simulink model "PoolofAdaptiveoscillatorsThree"  (R2019b)
settings: Solver=FixedStepAuto  StartTime=0.0  StopTime=t_sim  FixedStep=tsamp  MaxStep=0.01  RelTol=1e-3
values from neighbouring files (symbols this model uses):
  alpha_0_init = 0.01    [PoolofAdaptiveOscillatorsThree.m]
  alpha_init = 0    [PoolofAdaptiveOscillatorsThree.m]
  eta = 2    [AO_Oscillators.m]    (also in PoolofAdaptiveOscillatorsThree.m = 1)
  omega_init = 0    [PoolofAdaptiveOscillatorsThree.m]
  phi_init = 0    [PoolofAdaptiveOscillatorsThree.m]
  tsamp = T/100    (= 0.0125)    [AO_Oscillators.m]    (also in PoolofAdaptiveOscillatorsThree.m = 0.00625)
  v_omega = 13    [AO_Oscillators.m]    (also in PoolofAdaptiveOscillatorsThree.m = 2)
  v_phi = sqrt(24.2*v_omega)    [AO_Oscillators.m]    (also in PoolofAdaptiveOscillatorsThree.m = 2)
settings Model: Creator=dell  LastModifiedBy=dell

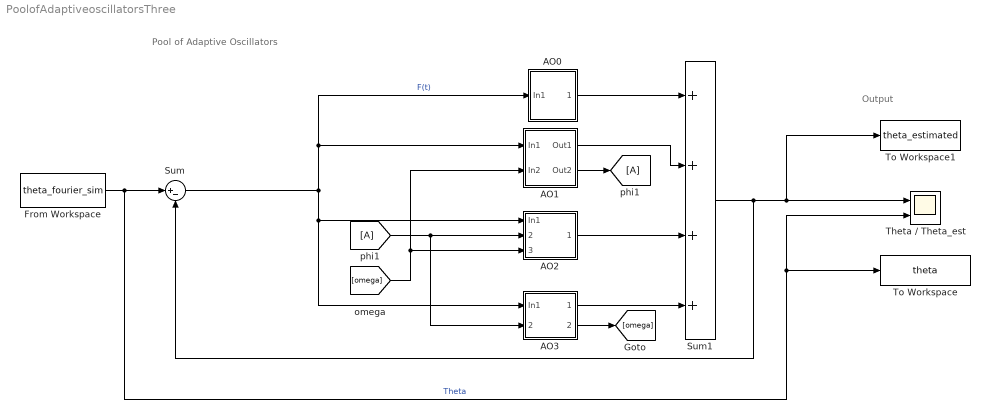
== system PoolofAdaptiveoscillatorsThree ==
  note: Pool of Adaptive Oscillators
  note: Output
  AO0 : Subsystem
      mask Display: image('F:\Masters\Thesis\Scripts\Images\integ.png'); % Use "Edit Image" on toolstrip to change.
  AO1 : Subsystem
      mask Display: image('F:\Masters\Thesis\Scripts\Images\ac symbol.png'); % Use "Edit Image" on toolstrip to change.
  AO2 : Subsystem
      mask Display: image('F:\Masters\Thesis\Scripts\Images\ac symbol.png'); % Use "Edit Image" on toolstrip to change.
  AO3 : Subsystem
      mask Display: image('F:\Masters\Thesis\Scripts\Images\ac symbol.png'); % Use "Edit Image" on toolstrip to change.
  From Workspace : FromWorkspace  VariableName=theta_fourier_sim  SampleTime=tsamp  Interpolate=off  OutputAfterFinalValue=Holding final value
  Sum : Sum  Inputs=|+-
  Sum1 : Sum  Inputs=4
  "Theta / Theta_est " : Scope  NumInputPorts=2
  To Workspace : ToWorkspace  VariableName=theta  SaveFormat=Timeseries  SampleTime=-1
  To Workspace1 : ToWorkspace  VariableName=theta_estimated  SaveFormat=Timeseries  SampleTime=-1
  wires:
  [A] -> AO3/2(Input), AO2/2(Input)
  AO1/2(Out2) -> [A]
  AO1/1(Out1) -> Sum1/2
  AO0/1(Out1) -> Sum1/1
  AO2/1(Out2) -> Sum1/3
  AO3/1(Out2) -> Sum1/4
  Sum/1 -> AO3/1(In1), AO2/1(In1), AO0/1(In1), AO1/1(In1)  "F(t)"
  From Workspace/1 -> "Theta / Theta_est "/2, To Workspace/1, Sum/1  "Theta"
  Sum1/1 -> Sum/2, "Theta / Theta_est "/1, To Workspace1/1
  AO3/2("omega ") -> [omega]
  [omega] -> AO1/2(In2), AO2/3("omega ")

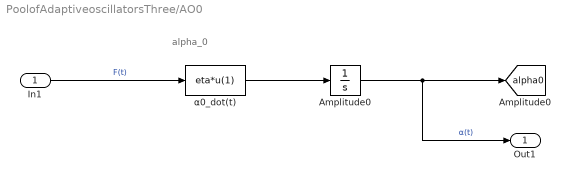
== system PoolofAdaptiveoscillatorsThree/AO0 ==
  note: alpha_0
  In1 : Inport
  Amplitude0 : Integrator  InitialCondition=alpha_0_init  ContinuousStateAttributes='Amplitude'
  α0_dot(t) : Fcn  Expr=eta*u(1)
  Out1 : Outport
  tag scope: alpha0=global
  wires:
  α0_dot(t)/1 -> Amplitude0/1
  Amplitude0/1 -> [alpha0], Out1/1  "α(t)"
  In1/1 -> α0_dot(t)/1  "F(t)"

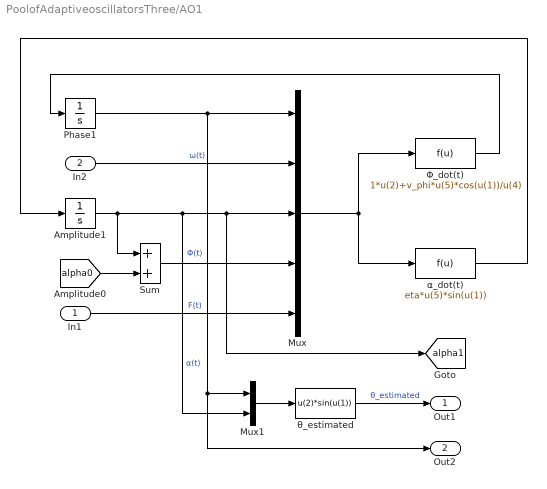
== system PoolofAdaptiveoscillatorsThree/AO1 ==
  In1 : Inport
  In2 : Inport  Port=2
  Amplitude1 : Integrator  InitialCondition=alpha_init  ContinuousStateAttributes='Amplitude'
  Mux : Mux  Inputs=5
  Mux1 : Mux  Inputs=2
  Phase1 : Integrator  InitialCondition=phi_init  ContinuousStateAttributes='Phase'
  Sum : Sum  Inputs=2
  Φ_dot(t) : Fcn  Expr=1*u(2)+v_phi*u(5)*cos(u(1))/u(4)
  α_dot(t) : Fcn  Expr=eta*u(5)*sin(u(1))
  θ_estimated : Fcn  Expr=u(2)*sin(u(1))
  Out1 : Outport
  Out2 : Outport  Port=2
  tag scope: alpha1=global
  wires:
  Mux/1 -> Φ_dot(t)/1, α_dot(t)/1
  α_dot(t)/1 -> Amplitude1/1
  Φ_dot(t)/1 -> Phase1/1
  Phase1/1 -> Out2/1, Mux1/1, Mux/1  "Φ(t)"
  Mux1/1 -> θ_estimated/1
  In2/1 -> Mux/2  "ω(t)"
  Amplitude1/1 -> Sum/1, Mux1/2, Mux/3, [alpha1]  "α(t)"
  [alpha0] -> Sum/2
  Sum/1 -> Mux/4
  In1/1 -> Mux/5  "F(t)"
  θ_estimated/1 -> Out1/1  "θ_estimated"

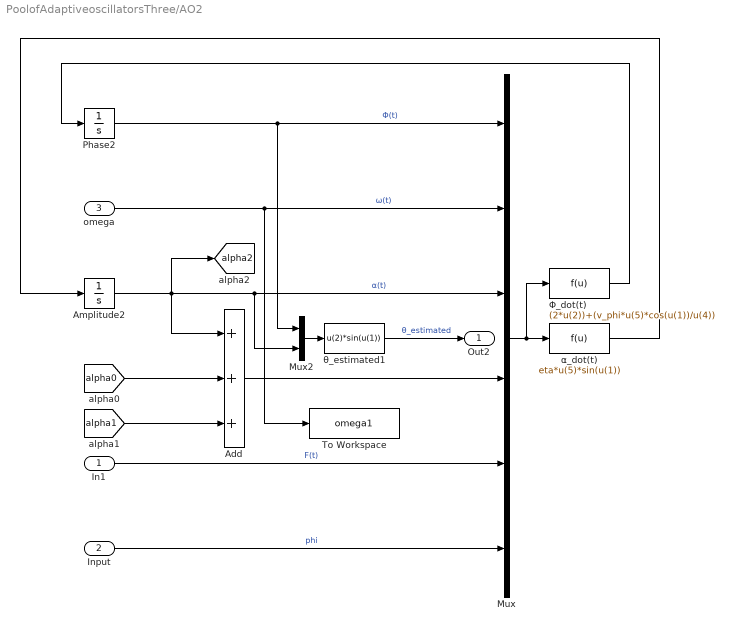
== system PoolofAdaptiveoscillatorsThree/AO2 ==
  In1 : Inport
  Input : Inport  Port=2
  "omega " : Inport  Port=3
  Add : Sum  Inputs=3
  Amplitude2 : Integrator  InitialCondition=alpha_init  ContinuousStateAttributes='Amplitude'
  Mux : Mux  Inputs=6
  Mux2 : Mux  Inputs=2
  Phase2 : Integrator  InitialCondition=phi_init  ContinuousStateAttributes='Phase'
  To Workspace : ToWorkspace  VariableName=omega1  SaveFormat=Structure With Time  SampleTime=-1
  Φ_dot(t) : Fcn  Expr=(2*u(2))+(v_phi*u(5)*cos(u(1))/u(4))
  α_dot(t) : Fcn  Expr=eta*u(5)*sin(u(1))
  θ_estimated1 : Fcn  Expr=u(2)*sin(u(1))
  Out2 : Outport
  tag scope: alpha2=global
  wires:
  Mux/1 -> α_dot(t)/1, Φ_dot(t)/1
  [alpha1] -> Add/3
  [alpha0] -> Add/2
  Phase2/1 -> Mux2/1, Mux/1  "Φ(t)"
  "omega "/1 -> To Workspace/1, Mux/2  "ω(t)"
  Φ_dot(t)/1 -> Phase2/1
  α_dot(t)/1 -> Amplitude2/1
  Input/1 -> Mux/6  "phi"
  In1/1 -> Mux/5  "F(t)"
  Add/1 -> Mux/4
  θ_estimated1/1 -> Out2/1  "θ_estimated"
  Mux2/1 -> θ_estimated1/1
  Amplitude2/1 -> Add/1, Mux2/2, Mux/3, [alpha2]  "α(t)"

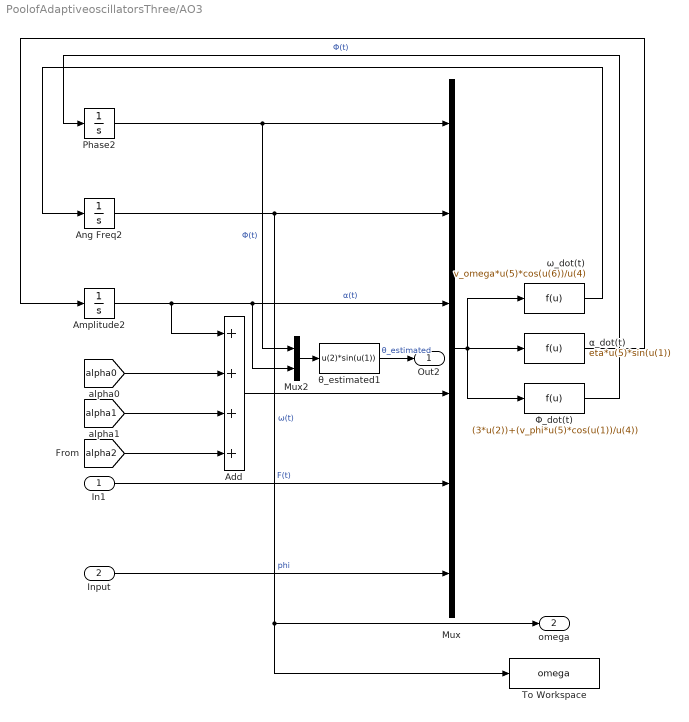
== system PoolofAdaptiveoscillatorsThree/AO3 ==
  In1 : Inport
  Input : Inport  Port=2
  Add : Sum  Inputs=4
  Amplitude2 : Integrator  InitialCondition=alpha_init  ContinuousStateAttributes='Amplitude'
  Ang Freq2 : Integrator  InitialCondition=omega_init  ContinuousStateAttributes='AngularFrequency'
  Mux : Mux  Inputs=6
  Mux2 : Mux  Inputs=2
  Phase2 : Integrator  InitialCondition=phi_init  ContinuousStateAttributes='Phase'
  To Workspace : ToWorkspace  VariableName=omega  SaveFormat=Structure With Time  SampleTime=-1
  Φ_dot(t) : Fcn  Expr=(3*u(2))+(v_phi*u(5)*cos(u(1))/u(4))
  α_dot(t) : Fcn  Expr=eta*u(5)*sin(u(1))
  θ_estimated1 : Fcn  Expr=u(2)*sin(u(1))
  ω_dot(t) : Fcn  Expr=v_omega*u(5)*cos(u(6))/u(4)
  Out2 : Outport
  "omega " : Outport  Port=2
  wires:
  ω_dot(t)/1 -> Ang Freq2/1
  Ang Freq2/1 -> "omega "/1, To Workspace/1, Mux/2  "ω(t)"
  Phase2/1 -> Mux2/1, Mux/1  "Φ(t)"
  α_dot(t)/1 -> Amplitude2/1
  Input/1 -> Mux/6  "phi"
  Amplitude2/1 -> Add/1, Mux2/2, Mux/3  "α(t)"
  Add/1 -> Mux/4
  In1/1 -> Mux/5  "F(t)"
  Mux/1 -> Φ_dot(t)/1, ω_dot(t)/1, α_dot(t)/1
  [alpha0] -> Add/2
  [alpha1] -> Add/3
  [alpha2] -> Add/4
  θ_estimated1/1 -> Out2/1  "θ_estimated"
  Mux2/1 -> θ_estimated1/1
  Φ_dot(t)/1 -> Phase2/1  "Φ(t)"
